simulink model "task11-Simulink"  (R2015b)
settings: Solver=ode23t  StartTime=0.0  StopTime=0.5  RelTol=1e-3
values from neighbouring files (symbols this model uses):
  A = [0 0 0 1 0 0;     0 0 0 0 1 0;      0 0 0 0 0 1;     (kt-ko)/J1 kt/(J1*n^2) -kt/J1 (dt-do)/J1 dt/(J1*n^2) -dt/J1;    -kt/(Jmg*n^2) -kt/((n^4)*Jmg) kt/((n^2)*Jmg) -dt/(Jmg*n^2) 1/Jmg*(-Km*Kemf/R-dt/(n^4)) dt/(n^2*Jmg);    kt/Jout kt/((n^2)*Jout) (-kt-kr)/Jout dt/Jout dt/((n^2)*Jout) -(dt+dj)/Jout]    [All Tasks Compiled.m]
  Acs = (pi/4)*(ds)^2    [All Tasks Compiled.m]
  B = [0 0 0 0 Km/(R*Jmg) 0]'    [All Tasks Compiled.m]
  C = eye(6)    [All Tasks Compiled.m]
  D = [0 0 0 0 0 0]'    [All Tasks Compiled.m]
  dj = dt    (= 1.5)    [All Tasks Compiled.m]
  ds = d-(13*sqrt(3)/24)*p    [All Tasks Compiled.m]
  kj = Acs*Esteel/L    [All Tasks Compiled.m]
  kr = kj*(p/(2*pi))^2    [All Tasks Compiled.m]
  mu = 0.2    [All Tasks Compiled.m]
  n2 = n^2    [All Tasks Compiled.m]
  p = 1.25/1000    (= 0.00125)    [All Tasks Compiled.m]
  T = 25    [All Tasks Compiled.m]
undefined symbols (not defined in the file or in its folder): sigbuilder_block
libraries: simulink x1
settings Model: Creator=atang  LastModifiedBy=atang
settings DataIOCC: LimitDataPoints=off

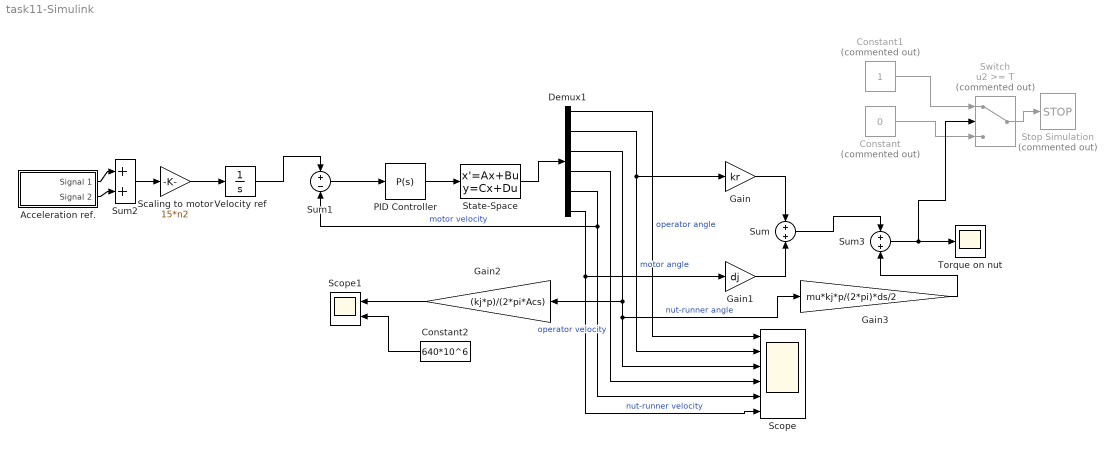
== system task11-Simulink ==
  Acceleration ref. : Subsystem  Tag=STV Subsys  LoadFcn=sigbuilder_block('load');  StartFcn=sigbuilder_block('start');  StopFcn=sigbuilder_block('stop');  ClipboardFcn=sigbuilder_block('clipboard');  mask(Sigbuilder block){}
      mask help: Sigbuilder GUI
      mask init:
      | if ~strcmp(get_param(bdroot(gcbh),'SimulationStatus'),'stopped') tuvar = sigbuilder_block('maskInit'); end
      settings: CopyFcn=sigbuilder_block('copy');  DeleteFcn=sigbuilder_block('delete');  ModelCloseFcn=sigbuilder_block('modelClose');  PreSaveFcn=sigbuilder_block('preSave');  PauseFcn=sigbuilder_block('pause')  ContinueFcn=sigbuilder_block('continue')  NameChangeFcn=sigbuilder_block('namechange');  OpenFcn=sigbuilder_block('open',[214.5 141.75 550.5 399.75 ]);  CloseFcn=sigbuilder_block('close');
      mask Display: plot(0,0,100,100,[10,10,40,40,10],[80,20,20,80,80],[40,10],[50,50], [40,27,10],[65,72,56],[40,25,25,10],[28,28,43,43]);
  Constant : Constant  Commented=on  Value=0
  Constant1 : Constant  Commented=on
  Constant2 : Constant  Value=640*10^6
  Demux1 : Demux  Outputs=6
  Gain : Gain  Gain=kr
  Gain1 : Gain  Gain=dj
  Gain2 : Gain  Gain=(kj*p)/(2*pi*Acs)
  Gain3 : Gain  Gain=mu*kj*p/(2*pi)*ds/2
  PID Controller : simulink/Continuous/PID Controller  Controller=P  TimeDomain=Continuous-time  SampleTime=-1  IntegratorMethod=Forward Euler  FilterMethod=Forward Euler  Form=Parallel  UseFilter=on  ControllerParametersSource=internal  P=8.5  I=10  D=0  N=100  InitialConditionSource=internal  InitialConditionForIntegrator=0  InitialConditionForFilter=0  ExternalReset=none  LimitOutput=off  UpperSaturationLimit=inf  LowerSaturationLimit=-inf  LinearizeAsGain=on  AntiWindupMode=none  Kb=1  TrackingMode=off  Kt=1  PParamMin=[]  PParamMax=[]  IParamMin=[]  IParamMax=[]  DParamMin=[]  DParamMax=[]  NParamMin=[]  NParamMax=[]  KbParamMin=[]  KbParamMax=[]  KtParamMin=[]  KtParamMax=[]  POutMin=[]  POutMax=[]  IOutMin=[]  IOutMax=[]  DOutMin=[]  DOutMax=[]  NOutMin=[]  NOutMax=[]  KbOutMin=[]  KbOutMax=[]  KtOutMin=[]  KtOutMax=[]  IntegratorOutMin=[]  IntegratorOutMax=[]  FilterOutMin=[]  FilterOutMax=[]  SumOutMin=[]  SumOutMax=[]  SumI1OutMin=[]  SumI1OutMax=[]  SumI2OutMin=[]  SumI2OutMax=[]  SumI3OutMin=[]  SumI3OutMax=[]  SumDOutMin=[]  SumDOutMax=[]  SaturationOutMin=[]  SaturationOutMax=[]  IntegratorContinuousStateAttributes=''  IntegratorStateMustResolveToSignalObject=off  IntegratorRTWStateStorageClass=Auto  FilterContinuousStateAttributes=''  FilterStateMustResolveToSignalObject=off  FilterRTWStateStorageClass=Auto  DifferentiatorICPrevScaledInput=0  DifferentiatorOutMin=[]  DifferentiatorOutMax=[]
  Scaling to motor : Gain  Gain=15*n2
  Scope : Scope  NumInputPorts=6
  Scope1 : Scope  NumInputPorts=2
  State-Space : StateSpace  A=A  B=B  C=C  D=D  X0=0
  Stop Simulation : Stop  Commented=on
  Sum : Sum
  Sum1 : Sum  Inputs=+-
  Sum2 : Sum  Inputs=|++
  Sum3 : Sum
  Switch : Switch  Commented=on  Threshold=T
  Torque on nut : Scope
  Velocity ref : Integrator
  wires:
  Demux1/2 -> Scope/2, Gain/1  "motor angle"
  Demux1/5 -> Scope/5, Sum1/2  "motor velocity"
  State-Space/1 -> Demux1/1
  Gain/1 -> Sum/1
  Gain1/1 -> Sum/2
  Sum/1 -> Sum3/1
  Acceleration ref./1(Signal 1) -> Sum2/1
  Acceleration ref./2(Signal 2) -> Sum2/2
  Sum2/1 -> Scaling to motor/1
  Scaling to motor/1 -> Velocity ref/1
  Switch/1 -> Stop Simulation/1
  Constant/1 -> Switch/3
  Constant1/1 -> Switch/1
  PID Controller/1 -> State-Space/1
  Sum1/1 -> PID Controller/1
  Velocity ref/1 -> Sum1/1
  Gain2/1 -> Scope1/1
  Constant2/1 -> Scope1/2
  Gain3/1 -> Sum3/2
  Sum3/1 -> Switch/2, Torque on nut/1
  Demux1/6 -> Scope/6, Gain1/1  "nut-runner velocity"
  Demux1/4 -> Scope/4  "operator velocity"
  Demux1/3 -> Gain2/1, Gain3/1, Scope/3  "nut-runner angle"
  Demux1/1 -> Scope/1  "operator angle"

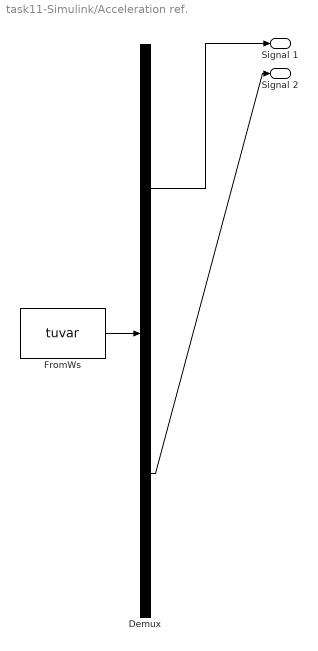
== system task11-Simulink/Acceleration ref. ==
  Demux : Demux  Tag=STV Demux  Outputs=2
  FromWs : FromWorkspace  Tag=STV FromWs  VariableName=tuvar  SampleTime=0
      SigBuilderData=|
      | common.afterFinalStr = 'Extrapolate'
      | common.sampleTime = 0
      | dataSet.timeRange = [0 10]
      | dataSet.name = 'Group 1'
      | sbobj.Groups.Name = 'Group 1'
      | sbobj.Groups.Signals(1).Name = 'Signal 1'
      | sbobj.Groups.Signals(1).XData = [0 0.2 0.2 10]
      | sbobj.Groups.Signals(1).YData = [1 1 0 0]
      | sbobj.Groups.Signals(2).Name = 'Signal 2'
      | sbobj.Groups.Signals(2).XData = [0 2.8 2.8 3 3 10]
      | sbobj.Groups.Signals(2).YData = [0 0 -1 -1 0 0]
  Signal 1 : Outport  Tag=STV Outport
  Signal 2 : Outport  Tag=STV Outport  Port=2
  wires:
  Demux/1 -> Signal 1/1
  FromWs/1 -> Demux/1
  Demux/2 -> Signal 2/1
